simulink model "thermal_model"  (R2026a)
settings: Solver=VariableStepAuto  StopTime=300
undefined symbols (not defined in the file): engine
settings Model: Creator=GOD  LastModifiedBy=GOD

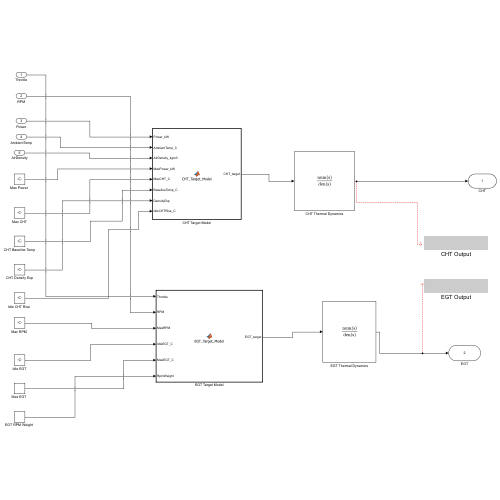
[thumbnail: Simulink's stored preview of the top-level diagram]
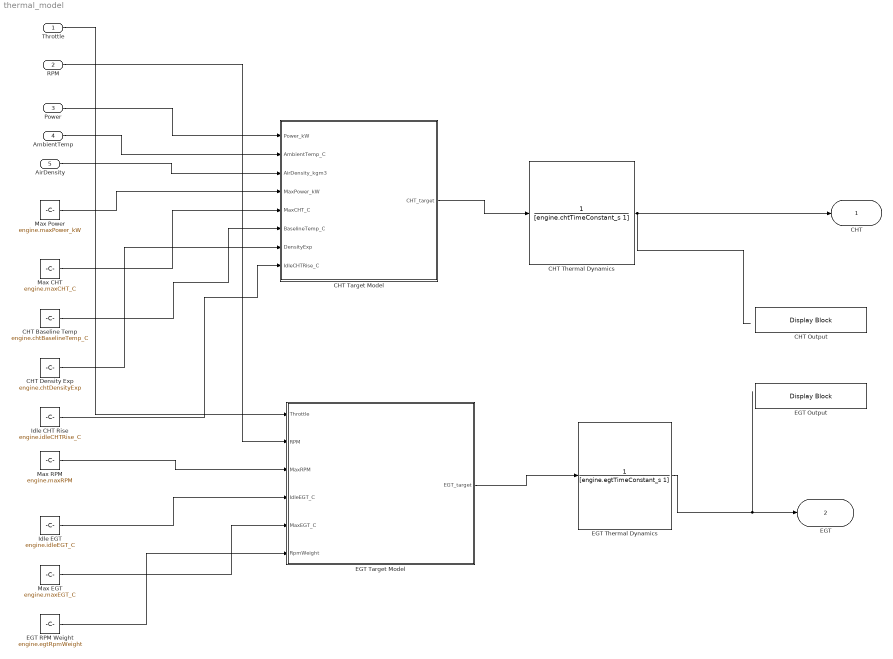
== system thermal_model ==
  Throttle : Inport
  RPM : Inport  Port=2
  Power : Inport  Port=3
  AmbientTemp : Inport  Port=4
  AirDensity : Inport  Port=5
  CHT Baseline Temp : Constant  Value=engine.chtBaselineTemp_C
  CHT Density Exp : Constant  Value=engine.chtDensityExp
  CHT Output : DisplayBlock  LabelPosition=Hide  Transparency=1  GridColor=[0.502, 0.502, 0.502]
  CHT Target Model : MATLAB Function  TreatAsAtomicUnit=on
  CHT Thermal Dynamics : TransferFcn  Denominator=[engine.chtTimeConstant_s 1]
  EGT Output : DisplayBlock  LabelPosition=Hide  Transparency=1  GridColor=[0.502, 0.502, 0.502]
  "EGT RPM Weight " : Constant  Value=engine.egtRpmWeight
  EGT Target Model : MATLAB Function  TreatAsAtomicUnit=on
  EGT Thermal Dynamics : TransferFcn  Denominator=[engine.egtTimeConstant_s 1]
  "Idle CHT Rise " : Constant  Value=engine.idleCHTRise_C
  Idle EGT : Constant  Value=engine.idleEGT_C
  Max CHT : Constant  Value=engine.maxCHT_C
  "Max EGT " : Constant  Value=engine.maxEGT_C
  "Max Power " : Constant  Value=engine.maxPower_kW
  "Max RPM " : Constant  Value=engine.maxRPM
  CHT : Outport
  EGT : Outport  Port=2
  wires:
  "Max Power "/1 -> CHT Target Model/4(MaxPower_kW)
  Max CHT/1 -> CHT Target Model/5(MaxCHT_C)
  CHT Baseline Temp/1 -> CHT Target Model/6(BaselineTemp_C)
  CHT Density Exp/1 -> CHT Target Model/7(DensityExp)
  "Idle CHT Rise "/1 -> CHT Target Model/8(IdleCHTRise_C)
  "Max RPM "/1 -> EGT Target Model/3(MaxRPM)
  Idle EGT/1 -> EGT Target Model/4(IdleEGT_C)
  "Max EGT "/1 -> EGT Target Model/5(MaxEGT_C)
  "EGT RPM Weight "/1 -> EGT Target Model/6(RpmWeight)
  CHT Target Model/1(CHT_target) -> CHT Thermal Dynamics/1
  EGT Target Model/1(EGT_target) -> EGT Thermal Dynamics/1
  CHT Thermal Dynamics/1 -> CHT/1
  EGT Thermal Dynamics/1 -> EGT/1
  Power/1 -> CHT Target Model/1(Power_kW)
  AmbientTemp/1 -> CHT Target Model/2(AmbientTemp_C)
  AirDensity/1 -> CHT Target Model/3(AirDensity_kgm3)
  Throttle/1 -> EGT Target Model/1(Throttle)
  RPM/1 -> EGT Target Model/2(RPM)

== matlab function thermal_model/EGT Target Model ==
  data: Throttle input; EGT_target output; RPM input; MaxRPM input; IdleEGT_C input; MaxEGT_C input; RpmWeight input
function EGT_target = EGT_Target_Model(Throttle, RPM, MaxRPM, IdleEGT_C, ...
    MaxEGT_C, RpmWeight)
% Engineering-assumption steady-state EGT target.
% EGT depends mainly on fuel/air mixture (approximated by throttle),
% with a secondary contribution from engine speed.
rpmFraction = RPM / MaxRPM;
if rpmFraction < 0
    rpmFraction = 0;
elseif rpmFraction > 1
    rpmFraction = 1;
end

throttleClipped = Throttle;
if throttleClipped < 0
    throttleClipped = 0;
elseif throttleClipped > 1
    throttleClipped = 1;
end

blend = RpmWeight * rpmFraction + (1 - RpmWeight) * throttleClipped;
EGT_target = IdleEGT_C + (MaxEGT_C - IdleEGT_C) * blend;
end

== matlab function thermal_model/CHT Target Model ==
  data: Power_kW input; CHT_target output; AmbientTemp_C input; AirDensity_kgm3 input; MaxPower_kW input; MaxCHT_C input; BaselineTemp_C input; DensityExp input; IdleCHTRise_C input
function CHT_target = CHT_Target_Model(Power_kW, AmbientTemp_C, AirDensity_kgm3, ...
    MaxPower_kW, MaxCHT_C, BaselineTemp_C, ...
    DensityExp, IdleCHTRise_C)
% Engineering-assumption steady-state CHT target.
% CHT rises with engine power output and falls with better cooling
% (higher air density = more effective convective cooling).
seaLevelDensity = 1.225;   % kg/m^3, ISA reference (physical constant)

powerFraction = Power_kW / MaxPower_kW;
if powerFraction < 0
    powerFraction = 0;
elseif powerFraction > 1
    powerFraction = 1;
end

coolingFactor = (seaLevelDensity / AirDensity_kgm3)^DensityExp;

CHT_target = AmbientTemp_C + IdleCHTRise_C + ...
    (MaxCHT_C - BaselineTemp_C - IdleCHTRise_C) * powerFraction * coolingFactor;
end
